simulink model "get_force_path"  (R2019b)
settings: Solver=VariableStepAuto  StartTime=0.0  StopTime=20  FixedStep=0.001  MaxStep=0.005  RelTol=1e-3
values from neighbouring files (symbols this model uses):
  g = 9.81    [simulation_setup.m]
  kxprop = 7    [simulation_setup.m]
  kzprop = 15    [simulation_setup.m]
  M = 1    [simulation_setup.m]
  m = 0.5    [simulation_setup.m]
  ts_planning = tun_chim_tun__obs_input.t(2) - tun_chim_tun__obs_input.t(1)    [simulation_setup.m]
settings Model: Creator=johan  LastModifiedBy=johan
settings DataIOCC: ReturnWorkspaceOutputs=off
settings DebuggingCC: ArithmeticOperatorsInVariantConditions=warning
settings SFSimCC: CustomCodeUndefinedFunction=UseInterfaceOnly

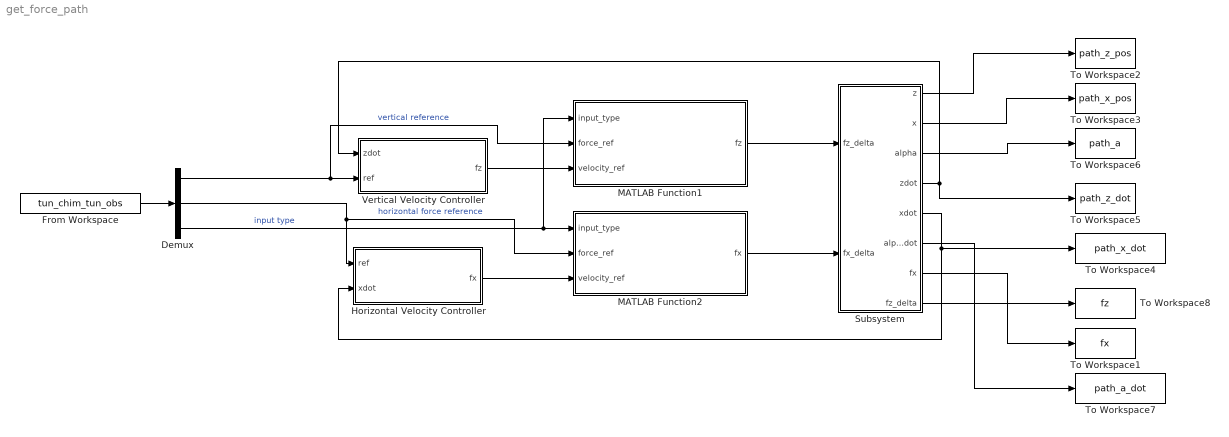
== system get_force_path ==
  Demux : Demux  Outputs=3
  From Workspace : FromWorkspace  VariableName=tun_chim_tun_obs  SampleTime=ts_planning  Interpolate=off  OutputAfterFinalValue=Holding final value
  Horizontal Velocity Controller : Subsystem
  MATLAB Function1 : MATLAB Function  TreatAsAtomicUnit=on
  MATLAB Function2 : MATLAB Function  TreatAsAtomicUnit=on
  Subsystem : Subsystem
  To Workspace1 : ToWorkspace  VariableName=fx  SaveFormat=Timeseries  SampleTime=-1
  To Workspace2 : ToWorkspace  VariableName=path_z_pos  SaveFormat=Timeseries  SampleTime=-1
  To Workspace3 : ToWorkspace  VariableName=path_x_pos  SaveFormat=Timeseries  SampleTime=-1
  To Workspace4 : ToWorkspace  VariableName=path_x_dot  SaveFormat=Timeseries  SampleTime=-1
  To Workspace5 : ToWorkspace  VariableName=path_z_dot  SaveFormat=Timeseries  SampleTime=-1
  To Workspace6 : ToWorkspace  VariableName=path_a  SaveFormat=Timeseries  SampleTime=-1
  To Workspace7 : ToWorkspace  VariableName=path_a_dot  SaveFormat=Timeseries  SampleTime=-1
  To Workspace8 : ToWorkspace  VariableName=fz  SaveFormat=Timeseries  SampleTime=-1
  Vertical Velocity Controller : Subsystem
  wires:
  MATLAB Function1/1(fz) -> Subsystem/1(fz_delta)
  MATLAB Function2/1(fx) -> Subsystem/2("fx_delta ")
  Subsystem/1(z) -> To Workspace2/1
  Subsystem/2(x) -> To Workspace3/1
  Subsystem/4(zdot) -> Vertical Velocity Controller/1(zdot), To Workspace5/1
  Subsystem/5(xdot) -> Horizontal Velocity Controller/2(xdot), To Workspace4/1
  From Workspace/1 -> Demux/1
  Demux/1 -> MATLAB Function1/2(force_ref), Vertical Velocity Controller/2(ref)  "vertical reference"
  Horizontal Velocity Controller/1(fx) -> MATLAB Function2/3(velocity_ref)
  Vertical Velocity Controller/1(fz) -> MATLAB Function1/3(velocity_ref)
  Demux/3 -> MATLAB Function1/1(input_type), MATLAB Function2/1(input_type)  "input type"
  Demux/2 -> Horizontal Velocity Controller/1(ref), MATLAB Function2/2(force_ref)  "horizontal force reference"
  Subsystem/7(fx) -> To Workspace1/1
  Subsystem/3(alpha) -> To Workspace6/1
  Subsystem/6(alphadot) -> To Workspace7/1
  Subsystem/8("fz_delta ") -> To Workspace8/1

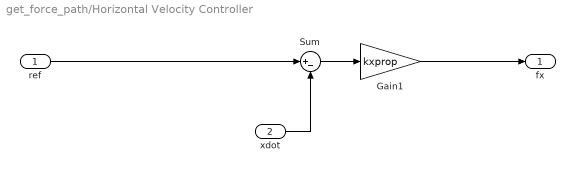
== system get_force_path/Horizontal Velocity Controller ==
  ref : Inport
  xdot : Inport  Port=2
  Gain1 : Gain  Gain=kxprop
  Sum : Sum  Inputs=|+-
  fx : Outport  VectorParamsAs1DForOutWhenUnconnected=off
  wires:
  Sum/1 -> Gain1/1
  ref/1 -> Sum/1
  xdot/1 -> Sum/2
  Gain1/1 -> fx/1

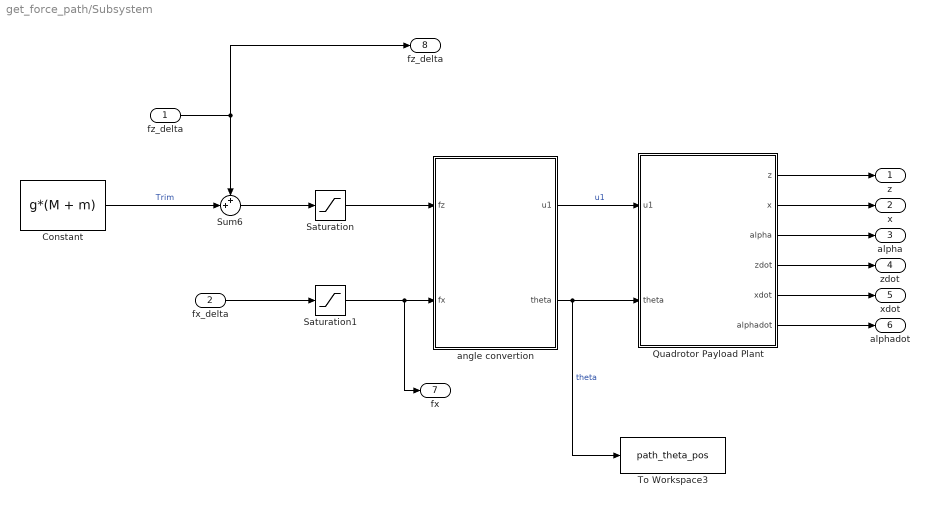
== system get_force_path/Subsystem ==
  fz_delta : Inport
  "fx_delta " : Inport  Port=2
  Constant : Constant  Value=g*(M + m)
  Quadrotor Payload Plant : Subsystem
  Saturation : Saturate  UpperLimit=3.5*(M+m)*g  LowerLimit=0
  Saturation1 : Saturate  UpperLimit=(M+m)*g*sin(pi/4)  LowerLimit=-(M+m)*g*sin(pi/4)
  Sum6 : Sum  Inputs=++|
  To Workspace3 : ToWorkspace  VariableName=path_theta_pos  SaveFormat=Timeseries  SampleTime=-1
  angle convertion : MATLAB Function  TreatAsAtomicUnit=on
  z : Outport  VectorParamsAs1DForOutWhenUnconnected=off
  x : Outport  Port=2  VectorParamsAs1DForOutWhenUnconnected=off
  alpha : Outport  Port=3  VectorParamsAs1DForOutWhenUnconnected=off
  zdot : Outport  Port=4  VectorParamsAs1DForOutWhenUnconnected=off
  xdot : Outport  Port=5  VectorParamsAs1DForOutWhenUnconnected=off
  alphadot : Outport  Port=6  VectorParamsAs1DForOutWhenUnconnected=off
  fx : Outport  Port=7  VectorParamsAs1DForOutWhenUnconnected=off
  "fz_delta " : Outport  Port=8  VectorParamsAs1DForOutWhenUnconnected=off
  wires:
  "fx_delta "/1 -> Saturation1/1
  fz_delta/1 -> Sum6/1, "fz_delta "/1
  Quadrotor Payload Plant/5(xdot) -> xdot/1
  Sum6/1 -> Saturation/1
  angle convertion/2(theta) -> To Workspace3/1, Quadrotor Payload Plant/2(theta)  "theta"
  angle convertion/1(u1) -> Quadrotor Payload Plant/1("u1 ")  "u1"
  Constant/1 -> Sum6/2  "Trim"
  Quadrotor Payload Plant/4(zdot) -> zdot/1
  Quadrotor Payload Plant/3(alpha) -> alpha/1
  Quadrotor Payload Plant/2(x) -> x/1
  Quadrotor Payload Plant/1(z) -> z/1
  Quadrotor Payload Plant/6(alphadot) -> alphadot/1
  Saturation/1 -> angle convertion/1(fz)
  Saturation1/1 -> fx/1, angle convertion/2(fx)

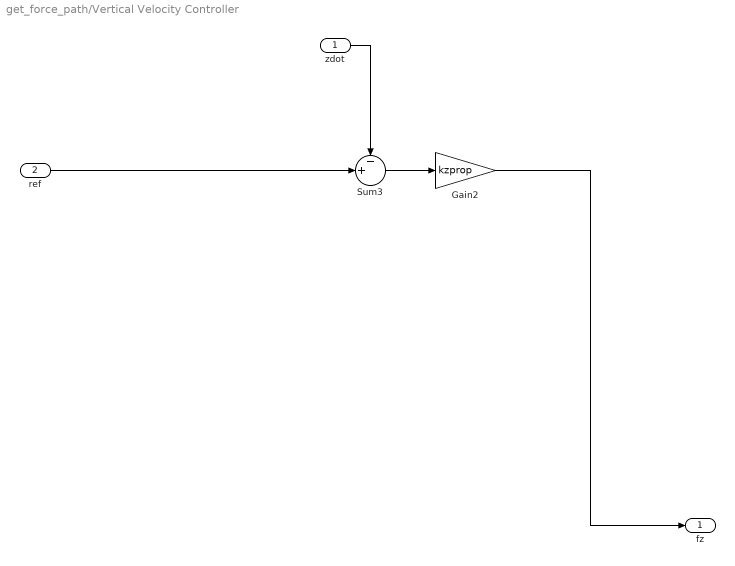
== system get_force_path/Vertical Velocity Controller ==
  zdot : Inport
  ref : Inport  Port=2
  Gain2 : Gain  Gain=kzprop
  Sum3 : Sum  Inputs=-+|
  fz : Outport  VectorParamsAs1DForOutWhenUnconnected=off
  wires:
  Sum3/1 -> Gain2/1
  zdot/1 -> Sum3/1
  ref/1 -> Sum3/2
  Gain2/1 -> fz/1

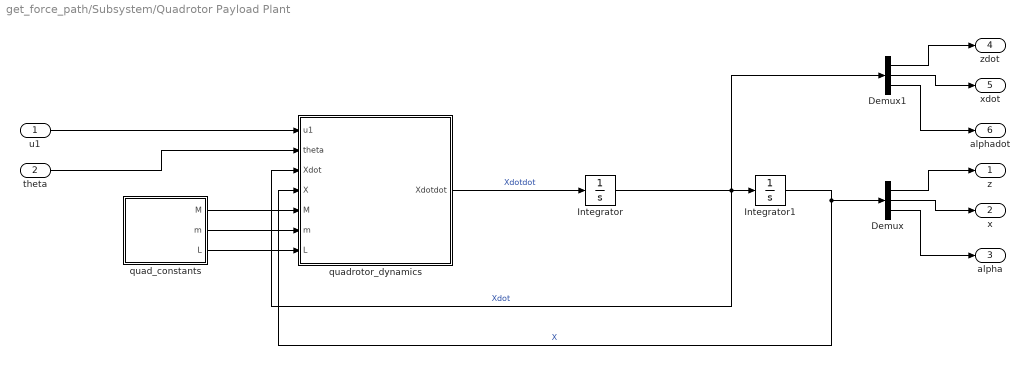
== system get_force_path/Subsystem/Quadrotor Payload Plant ==
  "u1 " : Inport
  theta : Inport  Port=2
  Demux : Demux  Outputs=3
  Demux1 : Demux  Outputs=3
  Integrator : Integrator  InitialCondition=[0 0 0]
  Integrator1 : Integrator  InitialCondition=[0 0 0]
  quad_constants : MATLAB Function  TreatAsAtomicUnit=on
  quadrotor_dynamics : MATLAB Function  TreatAsAtomicUnit=on
  z : Outport  VectorParamsAs1DForOutWhenUnconnected=off
  x : Outport  Port=2  VectorParamsAs1DForOutWhenUnconnected=off
  alpha : Outport  Port=3  VectorParamsAs1DForOutWhenUnconnected=off
  zdot : Outport  Port=4  VectorParamsAs1DForOutWhenUnconnected=off
  xdot : Outport  Port=5  VectorParamsAs1DForOutWhenUnconnected=off
  alphadot : Outport  Port=6  VectorParamsAs1DForOutWhenUnconnected=off
  wires:
  Integrator/1 -> quadrotor_dynamics/3(Xdot), Demux1/1, Integrator1/1  "Xdot"
  quad_constants/1(M) -> quadrotor_dynamics/5(M)
  Demux1/1 -> zdot/1
  Integrator1/1 -> Demux/1, quadrotor_dynamics/4(X)  "X"
  quadrotor_dynamics/1(Xdotdot) -> Integrator/1  "Xdotdot"
  Demux/1 -> z/1
  Demux/3 -> alpha/1
  Demux1/2 -> xdot/1
  Demux1/3 -> alphadot/1
  quad_constants/3(L) -> quadrotor_dynamics/7(L)
  quad_constants/2(m) -> quadrotor_dynamics/6(m)
  theta/1 -> quadrotor_dynamics/2(theta)
  "u1 "/1 -> quadrotor_dynamics/1(u1)
  Demux/2 -> x/1

== matlab function get_force_path/Subsystem/Quadrotor Payload Plant/quad_constants ==
  data: M output; m output; L output
function [M,m,L]= constants

M = 1;
m = 0.5;
L = 0.5;

== matlab function get_force_path/Subsystem/Quadrotor Payload Plant/quadrotor_dynamics ==
  data: u1 input; Xdotdot output; theta input; Xdot input; X input; M input; m input; L input

function Xdotdot = quadrotor_dynamics(u1, theta, Xdot, X, M, m, L)
g = 9.81;


alpha = X(3);
alphadot = Xdot(3);


fz = -g - ((m)/(M + m)) * L * cos(alpha )* alphadot^2;
fx = - (m/(M+m)) * L * sin(alpha )* alphadot^2;
gz = (1/(M + m)) * (cos(theta) + (m /(2 *M))* (cos(theta) - cos(theta - 2 * alpha)));
gx = (1/(M + m)) * (sin(theta) + (m /(2 *M))* (sin(theta) + sin(theta - 2 * alpha)));
ga = (1 / (M * L)) * sin(theta - alpha);

zdotdot = fz + gz*u1;
xdotdot = fx + gx*u1;
adotdot = ga*u1;

y = [zdotdot xdotdot adotdot];
Xdotdot = y;

== matlab function get_force_path/MATLAB Function1 ==
  data: input_type input; fz output; force_ref input; velocity_ref input
function fz = input_select(input_type,force_ref,velocity_ref)

fz = 0;
if (input_type == 0)
    fz = force_ref;
end
if (input_type == 1)
    fz = velocity_ref;
end
if (input_type == 2)
    fz = velocity_ref;
end

== matlab function get_force_path/Subsystem/angle convertion ==
  data: fz input; u1 output; fx input; theta output
function [u1,theta] = convert_inputs(fz,fx)
u1 = sqrt(fz^2 + fx^2);
theta = atan(fx/fz);

== matlab function get_force_path/MATLAB Function2 ==
  data: input_type input; fx output; force_ref input; velocity_ref input
function fx = input_select(input_type,force_ref,velocity_ref)

fx = 0;
if (input_type == 0)
    fx = force_ref;
end
if (input_type == 1)
    fx = velocity_ref;
end
if (input_type == 2)
    fx = velocity_ref;
end
